simulink model "exampleThermalNode_version1"  (Simulink 8.2)
settings: Solver=ode45  StartTime=0.0  StopTime=2*3600  RelTol=1e-3
libraries: carnot x1
settings Model: Creator=drhf  LastModifiedBy=drhf

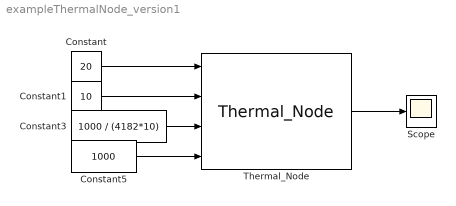
== system exampleThermalNode_version1 ==
  Constant : Constant  Value=20
  Constant1 : Constant  Value=10
  Constant3 : Constant  Value=1000 / (4182*10)
  Constant5 : Constant  Value=1000
  Scope : Scope
  Thermal_Node : carnot/Basic/Thermal_Models/Thermal_Node  UA=1  mcp=10*4182  cp_approx=4182  Tini=40
  wires:
  Thermal_Node/1 -> Scope/1
  Constant/1 -> Thermal_Node/1
  Constant1/1 -> Thermal_Node/2
  Constant3/1 -> Thermal_Node/3
  Constant5/1 -> Thermal_Node/4
